simulink model "Integrator_togler"  (R2024b)
settings: Solver=VariableStepAuto  StartTime=0.0  StopTime=10.0  RelTol=1e-3
undefined symbols (not defined in the file): DiscIntNeverNeededParam
libraries: simulink x1
settings Model: Creator=Emil  LastModifiedBy=Emil

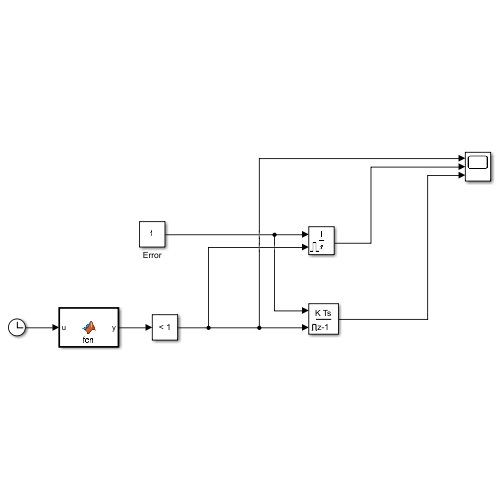
[thumbnail: Simulink's stored preview of the top-level diagram]
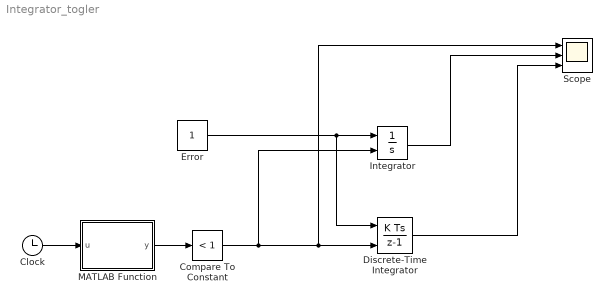
== system Integrator_togler ==
  Clock : Clock
  Compare To Constant : simulink/Logic and Bit Operations/Compare To Constant  relop=<  const=1  OutDataTypeStr=boolean
  Discrete-Time Integrator : DiscreteIntegrator  ExternalReset=level  SampleTime=-1  ICPrevOutput=DiscIntNeverNeededParam  ICPrevScaledInput=DiscIntNeverNeededParam
  Error : Constant
  Integrator : Integrator  ExternalReset=level
  MATLAB Function : MATLAB Function  TreatAsAtomicUnit=on
  Scope : Scope  NumInputPorts=3
  wires:
  Integrator/1 -> Scope/2
  Clock/1 -> MATLAB Function/1(u)
  Error/1 -> Discrete-Time Integrator/1, Integrator/1
  Discrete-Time Integrator/1 -> Scope/3
  MATLAB Function/1(y) -> Compare To Constant/1
  Compare To Constant/1 -> Integrator/2, Scope/1, Discrete-Time Integrator/2

== matlab function Integrator_togler/MATLAB Function ==
  data: u input; y output
function y = fcn(u)

if u <4
y = 1;
elseif u <8
    y=0.7;
else
    y=1;
end
